simulink model "blockredu"  (R2015a)
settings: Solver=ode45  StartTime=0.0  StopTime=10.0  RelTol=1e-3
settings Model: Creator=Prasad  LastModifiedBy=Prasad

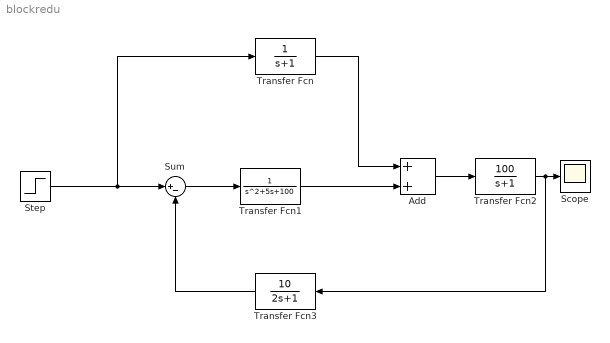
== system blockredu ==
  Add : Sum
  Scope : Scope
  Step : Step  SampleTime=0
  Sum : Sum  Inputs=|+-
  Transfer Fcn : TransferFcn  Denominator=[1 1]
  Transfer Fcn1 : TransferFcn  Denominator=[1 5 100]
  Transfer Fcn2 : TransferFcn  Numerator=[100]  Denominator=[1 1]
  Transfer Fcn3 : TransferFcn  Numerator=[10]  Denominator=[2 1]
  wires:
  Step/1 -> Transfer Fcn/1, Sum/1
  Sum/1 -> Transfer Fcn1/1
  Transfer Fcn1/1 -> Add/2
  Transfer Fcn/1 -> Add/1
  Add/1 -> Transfer Fcn2/1
  Transfer Fcn2/1 -> Transfer Fcn3/1, Scope/1
  Transfer Fcn3/1 -> Sum/2
